simulink model "a_half_bridge_average_value"  (R2025b)
settings: Solver=VariableStepAuto  StartTime=0.0  StopTime=5/60  RelTol=1e-3
libraries: fl_lib x14, nesl_utility x6
settings Model: SimulationMode=accelerator  Creator=gdudgeon  LastModifiedBy=gdudgeon

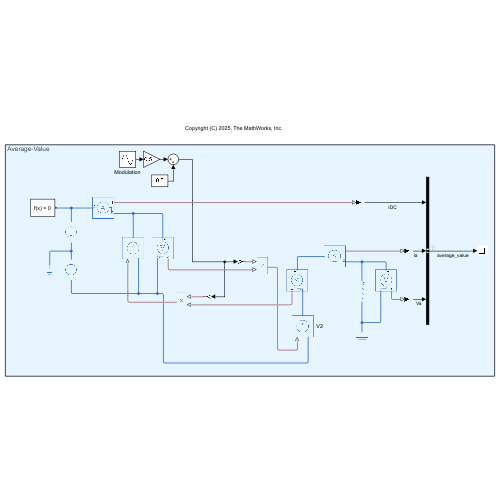
[thumbnail: Simulink's stored preview of the top-level diagram]
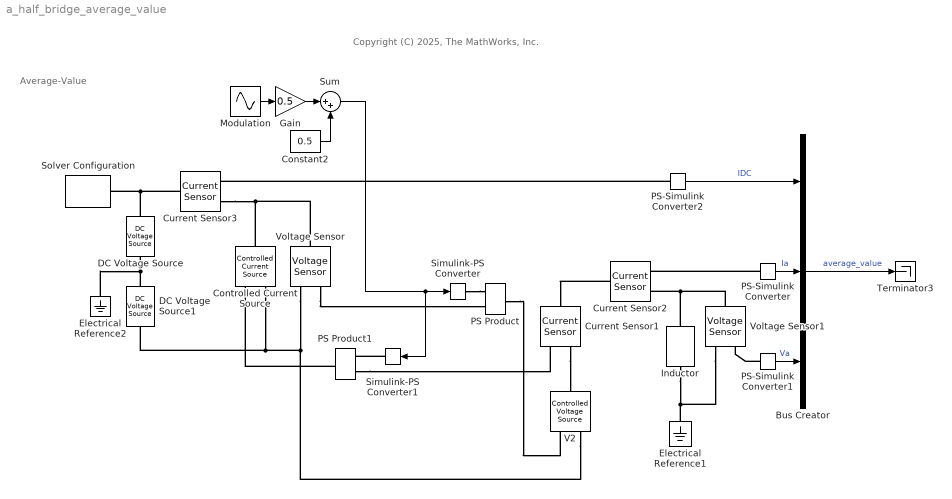
== system a_half_bridge_average_value ==
  note: Copyright (C) 2025, The MathWorks, Inc.
  note: Average-Value
  Bus Creator : BusCreator  Inputs=3
  Constant2 : Constant  Value=0.5  SampleTime=-1
  Controlled Current Source : fl_lib/Electrical/Electrical Sources/Controlled Current Source
  Current Sensor1 : fl_lib/Electrical/Electrical Sensors/Current Sensor
  Current Sensor2 : fl_lib/Electrical/Electrical Sensors/Current Sensor
  Current Sensor3 : fl_lib/Electrical/Electrical Sensors/Current Sensor
  DC Voltage Source : fl_lib/Electrical/Electrical Sources/DC Voltage Source  v0=50 V
  DC Voltage Source1 : fl_lib/Electrical/Electrical Sources/DC Voltage Source  v0=50 V
  Electrical Reference1 : fl_lib/Electrical/Electrical Elements/Electrical Reference
  Electrical Reference2 : fl_lib/Electrical/Electrical Elements/Electrical Reference
  Gain : Gain  Gain=0.5
  Inductor : fl_lib/Electrical/Electrical Elements/Inductor  l=0.01 H  r=1 Ohm  g=0 1/Ohm  i_specify=off  i_priority=None  i=0 A  i_nominal_specify=off  i_nominal_value=1  i_nominal_unit=A  v_specify=off  v_priority=High  v=0 V  v_nominal_specify=off  v_nominal_value=1  v_nominal_unit=V  i_L_specify=off  i_L_priority=High  i_L=0 A  i_L_nominal_specify=off  i_L_nominal_value=1  i_L_nominal_unit=A
  Modulation : Sin  Amplitude=0.8  Frequency=120*pi  SampleTime=0
  PS Product : fl_lib/Physical Signals/Functions/PS Product
  PS Product1 : fl_lib/Physical Signals/Functions/PS Product
  PS-Simulink Converter : nesl_utility/PS-Simulink Converter  PhysicalDomain=network_engine_domain  SubClassName=ps_output  LeftPortType=input  RightPortType=output  PseudoPeriodic=off  Frequencies=[]  VectorFormat=inherit  Unit=inherit  AffineConversion=off
  PS-Simulink Converter1 : nesl_utility/PS-Simulink Converter  PhysicalDomain=network_engine_domain  SubClassName=ps_output  LeftPortType=input  RightPortType=output  PseudoPeriodic=off  Frequencies=[]  VectorFormat=inherit  Unit=inherit  AffineConversion=off
  PS-Simulink Converter2 : nesl_utility/PS-Simulink Converter  PhysicalDomain=network_engine_domain  SubClassName=ps_output  LeftPortType=input  RightPortType=output  PseudoPeriodic=off  Frequencies=[]  VectorFormat=inherit  Unit=inherit  AffineConversion=off
  Simulink-PS Converter : nesl_utility/Simulink-PS Converter  PhysicalDomain=network_engine_domain  SubClassName=ps_input  LeftPortType=input  RightPortType=output  PseudoPeriodic=off  Frequencies=[]  NoiseDistribution=none  NoiseParameters=[]  Unit=1  AffineConversion=off  FilteringAndDerivatives=provide  SimscapeFilterOrder=1  InputFilterTimeConstant=0.001  UdotUserProvided=0
  Simulink-PS Converter1 : nesl_utility/Simulink-PS Converter  PhysicalDomain=network_engine_domain  SubClassName=ps_input  LeftPortType=input  RightPortType=output  PseudoPeriodic=off  Frequencies=[]  NoiseDistribution=none  NoiseParameters=[]  Unit=1  AffineConversion=off  FilteringAndDerivatives=provide  SimscapeFilterOrder=1  InputFilterTimeConstant=0.001  UdotUserProvided=0
  Solver Configuration : nesl_utility/Solver Configuration  PhysicalDomain=network_engine_domain  SubClassName=solver  LeftPortType=input  RightPortType=generic  Tones=[]  Harmonics=[]  SimulateNoise=off  Profile=off  UseLocalSampling=off  EnableSwitchedLinearOptims=on  FrequencyDomain=off  UseCCode=off  RelTol=0.001  AbsTol=0.001  MinStep=1e-09  ToWorkspace=off  RevertToSquareIcSolve=off  NumHomotopyIterations=100  PhasorMode=off  PhasorModeNumHarmonics=1  ConsistencySolver=NEWTON_XTOL_AFTER_FTOL  IndexReductionMethod=DerivativeReplacement  DoDC=off  ResidualTolerance=1e-09  ConsistencyTolSource=GLOBAL  ConsistencyAbsTol=0.001  ConsistencyRelTol=0.001  ConsistencyTolFactor=0.001  UseLocalSolver=on  LocalSolverChoice=NE_PARTITIONING_ADVANCER  ResolveIndetEquations=on  FunctionEvalNumThread=1  LocalSolverSampleTime=1e-6  DoFixedCost=off  MaxNonlinIter=3  MaxModeIter=2  ComputeImpulses=off  ImpulseIterations=2  LinearAlgebra=auto  LinearAlgebraNumThread=0  EquationFormulation=NE_TIME_EF  DelaysMemoryBudget=1024  AutomaticFiltering=off  FilteringTimeConstant=0.001  PartitionStorageMethod=AS_NEEDED  PartitionMemoryBudget=1024  PartitionMethod=ROBUST  MultibodyUseLocalSolver=off  MultibodyLocalSolverChoice=ODE1  MultibodyLocalSolverSampleTime=0.001
  Sum : Sum  Inputs=|++
  Terminator3 : Terminator
  V2 : fl_lib/Electrical/Electrical Sources/Controlled Voltage Source
  Voltage Sensor : fl_lib/Electrical/Electrical Sensors/Voltage Sensor
  Voltage Sensor1 : fl_lib/Electrical/Electrical Sensors/Voltage Sensor
  wires:
  PS-Simulink Converter/1 -> Bus Creator/2  "Ia"
  Sum/1 -> Simulink-PS Converter/1, Simulink-PS Converter1/1
  PS-Simulink Converter1/1 -> Bus Creator/3  "Va"
  Bus Creator/1 -> Terminator3/1  "average_value"
  PS-Simulink Converter2/1 -> Bus Creator/1  "IDC"
  Modulation/1 -> Gain/1
  Constant2/1 -> Sum/2
  Gain/1 -> Sum/1
  connections:
  Electrical Reference1/LConn1 -- Voltage Sensor1/RConn2 -- Inductor/RConn1
  DC Voltage Source/LConn1 -- Current Sensor3/LConn1 -- Solver Configuration/RConn1
  DC Voltage Source1/LConn1 -- Electrical Reference2/LConn1 -- DC Voltage Source/RConn1
  Controlled Current Source/RConn2 -- V2/RConn2 -- Voltage Sensor/RConn2 -- DC Voltage Source1/RConn1
  Current Sensor3/RConn2 -- Voltage Sensor/LConn1 -- Controlled Current Source/LConn1
  Current Sensor2/RConn2 -- Voltage Sensor1/LConn1 -- Inductor/LConn1
  PS-Simulink Converter2/LConn1 -- Current Sensor3/RConn1
  PS Product1/RConn1 -- Controlled Current Source/RConn1
  PS Product/RConn1 -- V2/RConn1
  Current Sensor1/RConn2 -- V2/LConn1
  PS-Simulink Converter/LConn1 -- Current Sensor2/RConn1
  Simulink-PS Converter1/RConn1 -- PS Product1/LConn2
  PS-Simulink Converter1/LConn1 -- Voltage Sensor1/RConn1
  Current Sensor2/LConn1 -- Current Sensor1/LConn1
  PS Product1/LConn1 -- Current Sensor1/RConn1
  Voltage Sensor/RConn1 -- PS Product/LConn2
  Simulink-PS Converter/RConn1 -- PS Product/LConn1
